simulink model "V2_4"  (R2023b)
settings: Solver=FixedStepAuto  StartTime=0.0  StopTime=inf  FixedStep=0.01  RelTol=1e-3
libraries: robotlib x14
settings Model: Creator=Renzhaofu  LastModifiedBy=Renzhaofu
settings OptimizationCC: EnhancedBackFolding=on  PassReuseOutputArgsAs=Individual arguments  ZeroExternalMemoryAtStartup=off  ZeroInternalMemoryAtStartup=off  MaxStackSize=64  OptimizeBlockOrder=speed  DifferentSizesBufferReuse=on  OptimizationCustomize=off  EfficientTunableParamExpr=on
settings DebuggingCC: ParameterTunabilityLossMsg=error
settings HardwareCC: ProdBitPerPointer=32  ProdBitPerSizeT=32  ProdBitPerPtrDiffT=32  ProdLargestAtomicFloat=None  ProdIntDivRoundTo=Undefined  ProdEndianess=Unspecified  ProdWordSize=32  ProdHWDeviceType=Generic->Unspecified (assume 32-bit Generic)
settings SFSimCC: MATLABDynamicMemAlloc=off
settings RTWCC: Description=Embedded Coder  SystemTargetFile=ert.tlc  HardwareBoard=Robot Operating System (ROS)  TLCOptions="-aInlineSetEventsForThisBaseRateFcn=TLC_FALSE -aSuppressMultiTaskScheduler=TLC_FALSE  -aRateBasedStepFcn=0"  TemplateMakefile=ert_default_tmf  Toolchain=Catkin  TargetLang=C++
settings CodeAppCC: ForceParamTrailComments=on  IgnoreCustomStorageClasses=off  OperatorAnnotations=on  SimulinkDataObjDesc=on  SFDataObjDesc=on  InsertBlockDesc=on

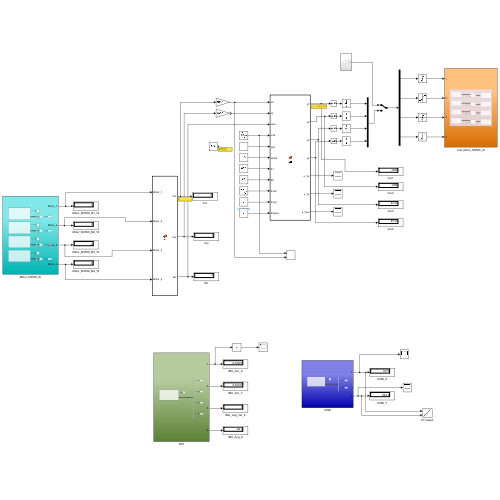
[thumbnail: Simulink's stored preview of the top-level diagram]
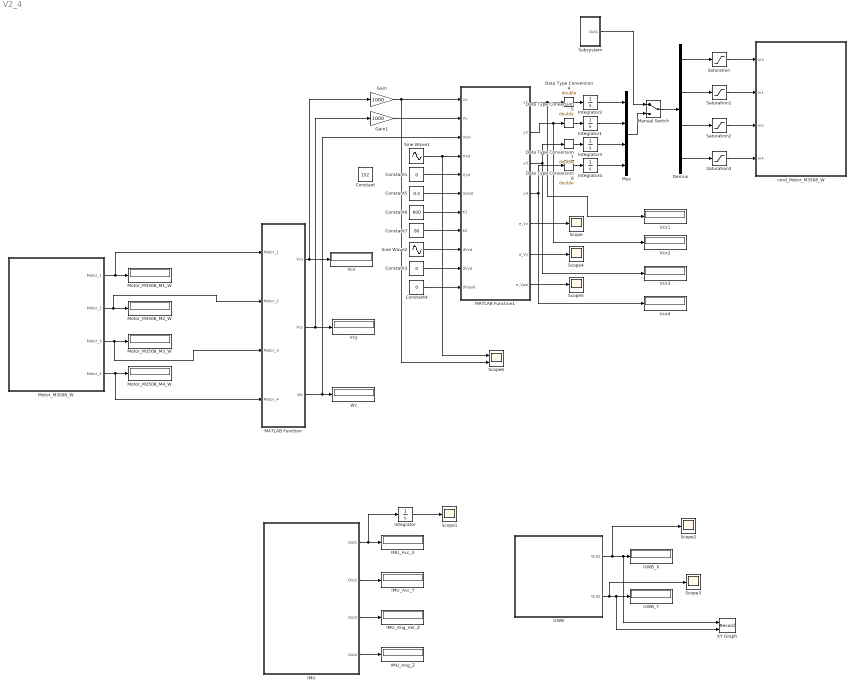
== system V2_4 ==
  Constant : Constant  Value=152
  Constant1 : Constant  Value=0
  Constant3 : Constant  Value=0
  Constant4 : Constant  Value=0
  Constant5 : Constant  Value=0.5
  Constant6 : Constant  Value=600
  Constant7 : Constant  Value=80
  Data Type Conversion{4..5,7..8} (4 alike) : DataTypeConversion  OutDataTypeStr=double  SaturateOnIntegerOverflow=off  RndMeth=Floor
  Demux : Demux
  Gain : Gain  Gain=1000
  Gain1 : Gain  Gain=1000
  IMU : Subsystem
  IMU_Acc_X : Display
  IMU_Acc_Y : Display
  IMU_Ang_Vel_Z : Display
  IMU_Ang_Z : Display
  Integrator{,1..4} (5 alike) : Integrator
  MATLAB Function : MATLAB Function  TreatAsAtomicUnit=on
  MATLAB Function1 : MATLAB Function  TreatAsAtomicUnit=on
  Manual Switch : ManualSwitch
  Motor_M3508_M1_W : Display
  Motor_M3508_M2_W : Display
  Motor_M3508_M3_W : Display
  Motor_M3508_M4_W : Display
  Motor_M3508_W : Subsystem
  Mux : Mux
  Saturation{,1..3} (4 alike) : Saturate  UpperLimit=500  LowerLimit=-500  OutDataTypeStr=single
  Scope{,1..5} (6 alike) : Scope
  Scope6 : Scope  NumInputPorts=2
  Sine Wave1 : Sin  Amplitude=152  Frequency=2*pi/5  SampleTime=0
  Sine Wave2 : Sin  Amplitude=152*2*pi/5  Frequency=2*pi/5  Phase=pi/2  SampleTime=0
  Subsystem : Subsystem
  UWB : Subsystem
  "UWB_X " : Display
  UWB_Y : Display
  Vcx{,1..4} (5 alike) : Display
  Vcy : Display
  Wc : Display
  XY Graph : Record  FileSettingsInternal="{\"entries\":[{\"content\":{\"excelSettings\":{\"content\":{},\"type\":\"Streamout.ExcelSettings\"}},\"type\":\"Streamout.FileSettingStorage\",\"uuid\":\"\"}],\"packageUris\":[\"http:\\/\\/schema.mathworks.com\\/mf0\\/streamout_blocks\\/R2020a\"],\"version\":\"1.0\"}"  Layout=[1 1]  SignalsInternal="{\"entries\":[{\"content\":{\"signals\":[{\"content\":{\"blockPath\":[],\"dimensions\":[1],\"domain\":\"\",\"lineColor\":\"#64d413\",\"port\":1,\"sid\":[\"\"],\"signalID\":2237,\"signalName\":\"UWB:1\"},\"type\":\"RecordBlkView.Signal\",\"uuid\":\"\"},{\"content\":{\"blockPath\":[],\"dimensions\":[1],\"domain\":\"\",\"lineColor\":\"#ff13a6\",\"port\":2,\"sid\":[\"\"],\"signalID\":2241,\"signalName\":\"UWB:2\"},\"type\":\"RecordBlkView.Signal\",\"uuid\":\"\"}]},\"type\":\"RecordBlkView.InputSignals\",\"uuid\":\"\"}],\"packageUris\":[\"http:\\/\\/schema.mathworks.com\\/mf0\\/streamout_blocks\\/R2020a\"],\"version\":\"1.0\"}"  VisualizationBindings="{\"xyplotplugin\":{\"info\":[{\"series\":[],\"subplotID\":1}]}}"  CompatibilityTag=XY
  cmd_Motor_M3508_W : Subsystem
  wires:
  Motor_M3508_W/1(Motor_1) -> MATLAB Function/1(Motor_1), Motor_M3508_M1_W/1
  Motor_M3508_W/4(Motor_4) -> MATLAB Function/4(Motor_4), Motor_M3508_M4_W/1
  IMU/1(Out1) -> Integrator/1, IMU_Acc_X/1
  IMU/2(Out2) -> IMU_Acc_Y/1
  IMU/3(Out3) -> IMU_Ang_Vel_Z/1
  IMU/4(Out4) -> IMU_Ang_Z/1
  UWB/1(Out1) -> Scope2/1, XY Graph/1, "UWB_X "/1
  UWB/2(Out2) -> Scope3/1, XY Graph/2, UWB_Y/1
  Motor_M3508_W/3(Motor_3) -> MATLAB Function/3(Motor_3), Motor_M3508_M3_W/1
  Motor_M3508_W/2(Motor_2) -> MATLAB Function/2(Motor_2), Motor_M3508_M2_W/1
  Integrator/1 -> Scope1/1
  MATLAB Function/1(Vcx) -> Gain/1, Vcx/1
  MATLAB Function/2(Vcy) -> Gain1/1, Vcy/1
  MATLAB Function/3(Wc) -> Wc/1, MATLAB Function1/3(Vpsi)
  Constant1/1 -> MATLAB Function1/5(Vyd)
  Sine Wave2/1 -> MATLAB Function1/9(dVxd)
  Constant3/1 -> MATLAB Function1/10(dVyd)
  Constant4/1 -> MATLAB Function1/11(dVpsid)
  Constant5/1 -> MATLAB Function1/6(Vpsid)
  Constant6/1 -> MATLAB Function1/7(K1)
  Constant7/1 -> MATLAB Function1/8(K2)
  MATLAB Function1/1(y1) -> Vcx1/1, Data Type Conversion4/1
  MATLAB Function1/2(y2) -> Vcx2/1, Data Type Conversion5/1
  MATLAB Function1/3(y3) -> Data Type Conversion7/1, Vcx3/1
  MATLAB Function1/4(y4) -> Vcx4/1, Data Type Conversion8/1
  Subsystem/1(Out1) -> Manual Switch/1
  Manual Switch/1 -> Demux/1
  Demux/1 -> Saturation/1
  Demux/2 -> Saturation1/1
  Demux/3 -> Saturation2/1
  Demux/4 -> Saturation3/1
  MATLAB Function1/5(e_Vx) -> Scope/1
  MATLAB Function1/6(e_Vy) -> Scope4/1
  MATLAB Function1/7(e_Vpsi) -> Scope5/1
  Saturation/1 -> cmd_Motor_M3508_W/1(In3)
  Saturation1/1 -> cmd_Motor_M3508_W/2(In1)
  Saturation2/1 -> cmd_Motor_M3508_W/3(In2)
  Saturation3/1 -> cmd_Motor_M3508_W/4(In4)
  Gain/1 -> Scope6/2, MATLAB Function1/1(Vx)
  Gain1/1 -> MATLAB Function1/2(Vy)
  Mux/1 -> Manual Switch/2
  Integrator3/1 -> Mux/3
  Integrator1/1 -> Mux/2
  Integrator2/1 -> Mux/1
  Integrator4/1 -> Mux/4
  Data Type Conversion4/1 -> Integrator2/1
  Data Type Conversion5/1 -> Integrator1/1
  Data Type Conversion7/1 -> Integrator3/1
  Data Type Conversion8/1 -> Integrator4/1
  Sine Wave1/1 -> Scope6/1, MATLAB Function1/4(Vxd)

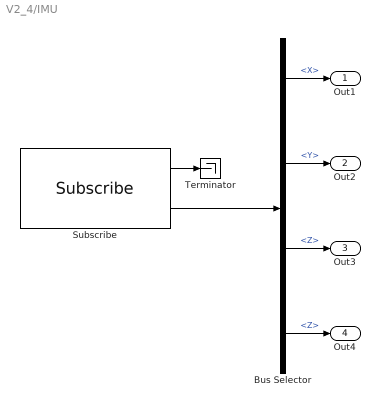
== system V2_4/IMU ==
  Bus Selector : BusSelector  OutputSignals=LinearAcceleration.X,LinearAcceleration.Y,AngularVelocity.Z,Orientation.Z
  Subscribe : robotlib/Subscribe  topicSource=Select from ROS network  topic=/IMU_Topic  messageType=sensor_msgs/Imu  SampleTime=0.1  legacyBusStruct=off  messageQueueLength=1
  Terminator : Terminator
  Out1 : Outport
  Out2 : Outport  Port=2
  Out3 : Outport  Port=3
  Out4 : Outport  Port=4
  wires:
  Bus Selector/3 -> Out3/1  "<Z>"
  Subscribe/2 -> Bus Selector/1
  Subscribe/1 -> Terminator/1
  Bus Selector/4 -> Out4/1  "<Z>"
  Bus Selector/2 -> Out2/1  "<Y>"
  Bus Selector/1 -> Out1/1  "<X>"

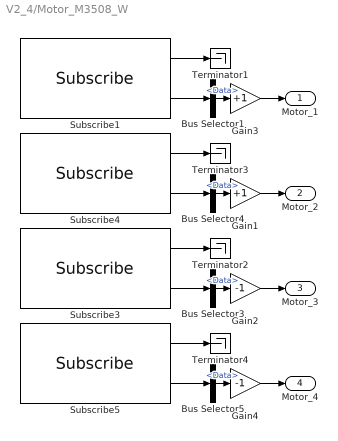
== system V2_4/Motor_M3508_W ==
  Bus Selector{1,3..5} (4 alike) : BusSelector  OutputSignals=Data
  Gain1 : Gain  Gain=+1
  Gain2 : Gain  Gain=-1
  Gain3 : Gain  Gain=+1
  Gain4 : Gain  Gain=-1
  Subscribe1 : robotlib/Subscribe  topicSource=Select from ROS network  topic=/Motor_M3508_M1_W_Topic  messageType=std_msgs/Float32  SampleTime=0.01  legacyBusStruct=off  messageQueueLength=1
  Subscribe3 : robotlib/Subscribe  topicSource=Select from ROS network  topic=/Motor_M3508_M3_W_Topic  messageType=std_msgs/Float32  SampleTime=0.01  legacyBusStruct=off  messageQueueLength=1
  Subscribe4 : robotlib/Subscribe  topicSource=Select from ROS network  topic=/Motor_M3508_M2_W_Topic  messageType=std_msgs/Float32  SampleTime=0.01  legacyBusStruct=off  messageQueueLength=1
  Subscribe5 : robotlib/Subscribe  topicSource=Select from ROS network  topic=/Motor_M3508_M4_W_Topic  messageType=std_msgs/Float32  SampleTime=0.01  legacyBusStruct=off  messageQueueLength=1
  Terminator{1..4} (4 alike) : Terminator
  Motor_1 : Outport
  Motor_2 : Outport  Port=2
  Motor_3 : Outport  Port=3
  Motor_4 : Outport  Port=4
  wires:
  Subscribe5/2 -> Bus Selector5/1
  Subscribe1/1 -> Terminator1/1
  Subscribe1/2 -> Bus Selector1/1
  Subscribe3/1 -> Terminator2/1
  Subscribe4/1 -> Terminator3/1
  Subscribe4/2 -> Bus Selector4/1
  Subscribe3/2 -> Bus Selector3/1
  Subscribe5/1 -> Terminator4/1
  Gain3/1 -> Motor_1/1
  Bus Selector1/1 -> Gain3/1  "<Data>"
  Bus Selector5/1 -> Gain4/1  "<Data>"
  Bus Selector3/1 -> Gain2/1  "<Data>"
  Bus Selector4/1 -> Gain1/1  "<Data>"
  Gain1/1 -> Motor_2/1
  Gain2/1 -> Motor_3/1
  Gain4/1 -> Motor_4/1

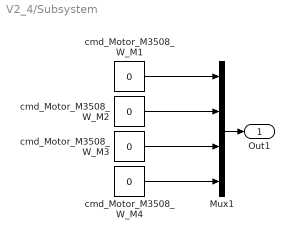
== system V2_4/Subsystem ==
  Mux1 : Mux
  cmd_Motor_M3508_W_M{1..4} (4 alike) : Constant  Value=0  OutDataTypeStr=single
  Out1 : Outport
  wires:
  cmd_Motor_M3508_W_M2/1 -> Mux1/2
  cmd_Motor_M3508_W_M3/1 -> Mux1/3
  cmd_Motor_M3508_W_M4/1 -> Mux1/4
  cmd_Motor_M3508_W_M1/1 -> Mux1/1
  Mux1/1 -> Out1/1

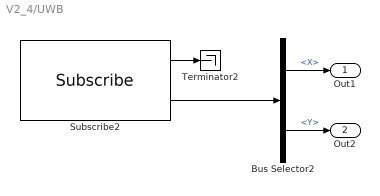
== system V2_4/UWB ==
  Bus Selector2 : BusSelector  OutputSignals=X,Y
  Subscribe2 : robotlib/Subscribe  topicSource=Select from ROS network  topic=/UWB_Topic  messageType=geometry_msgs/Point  SampleTime=0.1  legacyBusStruct=off  messageQueueLength=1
  Terminator2 : Terminator
  Out1 : Outport
  Out2 : Outport  Port=2
  wires:
  Bus Selector2/1 -> Out1/1  "<X>"
  Subscribe2/2 -> Bus Selector2/1
  Subscribe2/1 -> Terminator2/1
  Bus Selector2/2 -> Out2/1  "<Y>"

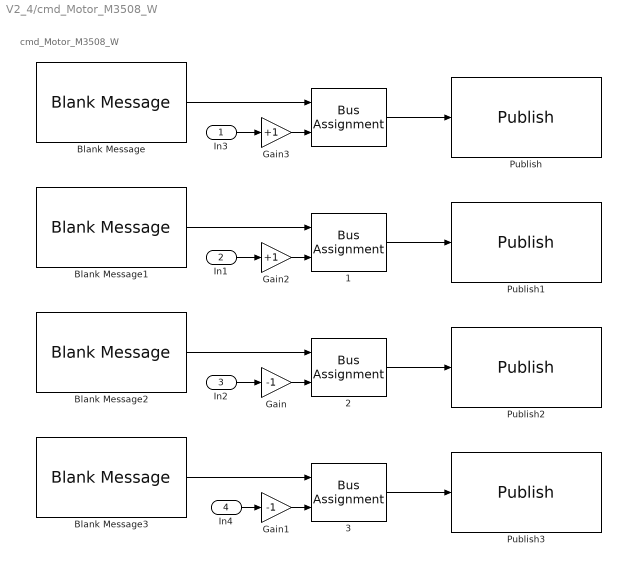
== system V2_4/cmd_Motor_M3508_W ==
  note: cmd_Motor_M3508_W
  In3 : Inport
  In1 : Inport  Port=2
  In2 : Inport  Port=3
  In4 : Inport  Port=4
   {,1..3} (4 alike) : BusAssignment  AssignedSignals=Data
  Blank Message{,1..3} (4 alike) : robotlib/Blank Message  messageClass=Message  entityType=std_msgs/Float32  messageType=std_msgs/Float32  SampleTime=inf  legacyBusStruct=off
  Gain : Gain  Gain=-1
  Gain1 : Gain  Gain=-1
  Gain2 : Gain  Gain=+1
  Gain3 : Gain  Gain=+1
  Publish : robotlib/Publish  topicSource=Select from ROS network  topic=/cmd_Motor_M3508_M1_W  messageType=std_msgs/Float32  legacyBusStruct=off  messageQueueLength=1
  Publish1 : robotlib/Publish  topicSource=Select from ROS network  topic=/cmd_Motor_M3508_M2_W  messageType=std_msgs/Float32  legacyBusStruct=off  messageQueueLength=1
  Publish2 : robotlib/Publish  topicSource=Select from ROS network  topic=/cmd_Motor_M3508_M3_W  messageType=std_msgs/Float32  legacyBusStruct=off  messageQueueLength=1
  Publish3 : robotlib/Publish  topicSource=Select from ROS network  topic=/cmd_Motor_M3508_M4_W  messageType=std_msgs/Float32  legacyBusStruct=off  messageQueueLength=1
  wires:
  Blank Message/1 -> " "/1
  " 3"/1 -> Publish3/1
  " 2"/1 -> Publish2/1
  In3/1 -> Gain3/1
  Gain2/1 -> " 1"/2
  Blank Message3/1 -> " 3"/1
  " "/1 -> Publish/1
  Blank Message2/1 -> " 2"/1
  In2/1 -> Gain/1
  Gain/1 -> " 2"/2
  Gain3/1 -> " "/2
  " 1"/1 -> Publish1/1
  Blank Message1/1 -> " 1"/1
  In1/1 -> Gain2/1
  Gain1/1 -> " 3"/2
  In4/1 -> Gain1/1

== matlab function V2_4/MATLAB Function1 ==
  data: Vx input; y1 output; Vy input; Vpsi input; y2 output; y3 output; Vxd input; Vyd input; Vpsid input; y4 output; K1 input; K2 input; dVxd input; dVyd input; dVpsid input; e_Vx output; e_Vy output; e_Vpsi output
function [y1, y2, y3, y4, e_Vx, e_Vy, e_Vpsi] = fcn(Vx, Vy, Vpsi, Vxd, Vyd, Vpsid, K1, K2, dVxd, dVyd, dVpsid)

Mec_Wheel_R = 152;
Mec_Wheeltrack = 150;
Mec_Wheelbase = 125;


phi_star = [+1 -1 -(Mec_Wheeltrack+Mec_Wheelbase);
            +1 +1 -(Mec_Wheeltrack+Mec_Wheelbase);
            +1 -1 +(Mec_Wheeltrack+Mec_Wheelbase);
            +1 +1 +(Mec_Wheeltrack+Mec_Wheelbase);];
% phi_star_trans = (1/60) .* phi_star;
phi_star_trans = (1/1) .* phi_star;

e_Vx = Vx - Vxd;
e_Vy = Vy - Vyd;
e_Vpsi = Vpsi - Vpsid;
e = [e_Vx;e_Vy;e_Vpsi];

dVd = [dVxd;dVyd;dVpsid];

u = -(1/Mec_Wheel_R) .* phi_star_trans * (K1*e + K2*sign(e) + dVd);

y1 = u(1);
y2 = u(2);
y3 = u(3);
y4 = u(4);

== matlab function V2_4/MATLAB Function ==
  data: Motor_1 input; Vcx output; Motor_2 input; Motor_3 input; Vcy output; Wc output; Motor_4 input
function [Vcx, Vcy, Wc] = fcn(Motor_1, Motor_2, Motor_3, Motor_4)

Mec_Wheel_R = 0.152;
Mec_Wheeltrack = 0.150;
Mec_Wheelbase = 0.125;

Robot_Vcx = Mec_Wheel_R / 4 * ((+Motor_1) + (+Motor_2) + (+Motor_3) + (+Motor_4)) / 60;
Robot_Vcy = Mec_Wheel_R / 4 * ((-Motor_1) + (+Motor_2) + (-Motor_3) + (+Motor_4)) / 60;
Robot_Wc  = Mec_Wheel_R / 4 * ((-Motor_1) + (-Motor_2) + (+Motor_3) + (+Motor_4)) / 60 / ((Mec_Wheeltrack + Mec_Wheelbase));

Vcx = Robot_Vcx;
Vcy = Robot_Vcy;
Wc =Robot_Wc;
